simulink model "PROJECTQ3"  (R2022a)
settings: Solver=VariableStepAuto  StartTime=0.0  StopTime=10.0  RelTol=1e-3
settings Model: Creator=1234567890  LastModifiedBy=1234567890

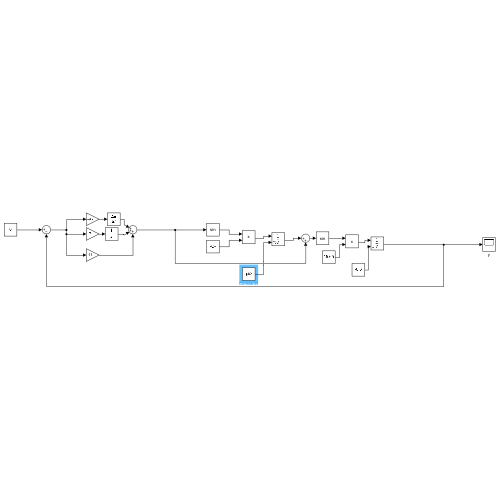
[thumbnail: Simulink's stored preview of the top-level diagram]
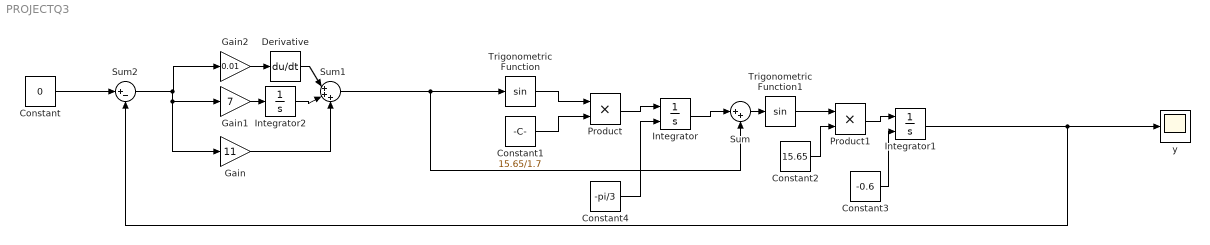
== system PROJECTQ3 ==
  Constant : Constant  Value=0
  Constant1 : Constant  Value=15.65/1.7
  Constant2 : Constant  Value=15.65
  Constant3 : Constant  Value=-0.6
  Constant4 : Constant  Value=-pi/3
  Derivative : Derivative
  Gain : Gain  Gain=11
  Gain1 : Gain  Gain=7
  Gain2 : Gain  Gain=0.01
  Integrator : Integrator  InitialConditionSource=external
  Integrator1 : Integrator  InitialConditionSource=external
  Integrator2 : Integrator
  Product : Product
  Product1 : Product
  Sum : Sum  Inputs=|++
  Sum1 : Sum  Inputs=|+++
  Sum2 : Sum  Inputs=|+-
  Trigonometric Function : Trigonometry
  Trigonometric Function1 : Trigonometry
  y : Scope
  wires:
  Constant1/1 -> Product/2
  Trigonometric Function/1 -> Product/1
  Product/1 -> Integrator/1
  Integrator/1 -> Sum/1
  Sum/1 -> Trigonometric Function1/1
  Trigonometric Function1/1 -> Product1/1
  Constant2/1 -> Product1/2
  Product1/1 -> Integrator1/1
  Integrator1/1 -> Sum2/2, y/1
  Gain/1 -> Sum1/3
  Gain2/1 -> Derivative/1
  Gain1/1 -> Integrator2/1
  Derivative/1 -> Sum1/1
  Integrator2/1 -> Sum1/2
  Sum1/1 -> Sum/2, Trigonometric Function/1
  Constant3/1 -> Integrator1/2
  Constant/1 -> Sum2/1
  Sum2/1 -> Gain/1, Gain1/1, Gain2/1
  Constant4/1 -> Integrator/2
